simulink model "Control_simulation"  (R2016a)
settings: Solver=ode4  StartTime=0.0  StopTime=200  FixedStep=0.001  MaxStep=0.01  RelTol=1e-6
values from neighbouring files (symbols this model uses):
  float =     [waveglider.mat]
  floatABC =     [waveglider.mat]
  gliderABC =     [waveglider.mat]
undefined symbols (not defined in the file or in its folder): magnitude, RAO_Vel, sigbuilder_block
libraries: simulink_extras x8, simulink x5, marine_gnc x4, fuzblock x1, marine_hydro x1
(part 1 of 3)
settings Model: Creator=Administrator  LastModifiedBy=DELL

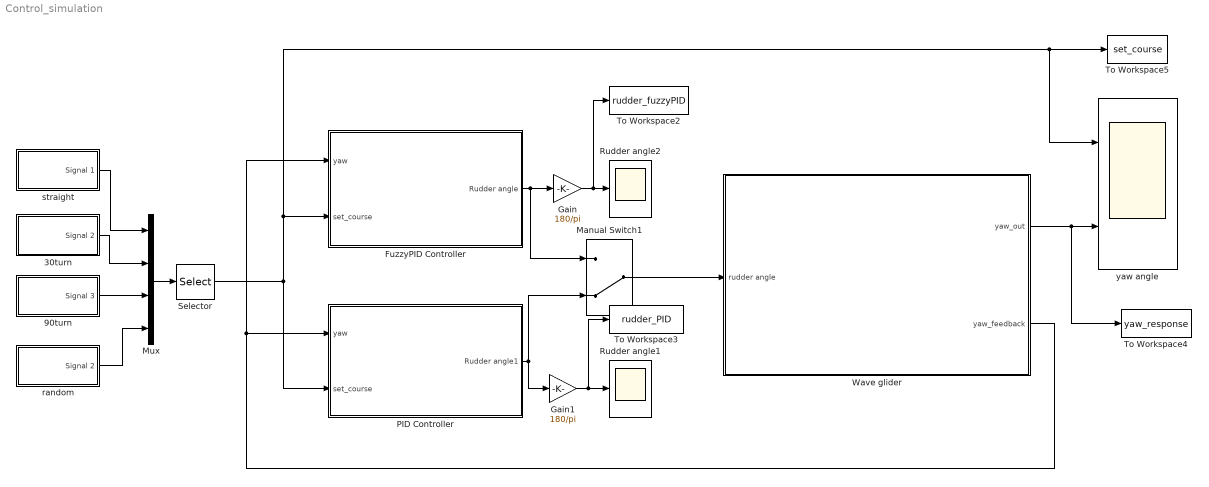
== system Control_simulation ==
  " yaw angle" : Scope  NumInputPorts=2
  30turn : Subsystem  Tag=STV Subsys  LoadFcn=sigbuilder_block('load');  StartFcn=sigbuilder_block('start');  StopFcn=sigbuilder_block('stop');  ClipboardFcn=sigbuilder_block('clipboard');  mask(Sigbuilder block){}
      mask help: Simulink:masks:SigbuilderBlock_MD
      mask init:
      | if ~strcmp(get_param(bdroot(gcbh),'SimulationStatus'),'stopped') tuvar = sigbuilder_block('maskInit'); end
      settings: CopyFcn=sigbuilder_block('copy');  DeleteFcn=sigbuilder_block('delete');  ModelCloseFcn=sigbuilder_block('modelClose');  PreSaveFcn=sigbuilder_block('preSave');  PauseFcn=sigbuilder_block('pause');  ContinueFcn=sigbuilder_block('continue');  NameChangeFcn=sigbuilder_block('namechange');  OpenFcn=sigbuilder_block('open',[6 105.75 1012.5 406.5 ]);  CloseFcn=sigbuilder_block('close');
      mask Display: plot(0, 0, 100, 100,[2, 2, 32, 32, 2], [68, 8, 8, 68, 68],[32, 2], [38, 38], [32, 19, 2],[53, 60, 44], [32, 17, 17, 2],[16, 16, 31, 31]);txt = getActiveGroup(gcbh);text(2, 100, txt,'verticalAlignment', 'top');
  90turn : Subsystem  Tag=STV Subsys  LoadFcn=sigbuilder_block('load');  StartFcn=sigbuilder_block('start');  StopFcn=sigbuilder_block('stop');  ClipboardFcn=sigbuilder_block('clipboard');  mask(Sigbuilder block){}
      mask help: Simulink:masks:SigbuilderBlock_MD
      mask init:
      | if ~strcmp(get_param(bdroot(gcbh),'SimulationStatus'),'stopped') tuvar = sigbuilder_block('maskInit'); end
      settings: CopyFcn=sigbuilder_block('copy');  DeleteFcn=sigbuilder_block('delete');  ModelCloseFcn=sigbuilder_block('modelClose');  PreSaveFcn=sigbuilder_block('preSave');  PauseFcn=sigbuilder_block('pause');  ContinueFcn=sigbuilder_block('continue');  NameChangeFcn=sigbuilder_block('namechange');  OpenFcn=sigbuilder_block('open',[6 16.5 1012.5 340.5 ]);  CloseFcn=sigbuilder_block('close');
      mask Display: plot(0, 0, 100, 100,[2, 2, 32, 32, 2], [68, 8, 8, 68, 68],[32, 2], [38, 38], [32, 19, 2],[53, 60, 44], [32, 17, 17, 2],[16, 16, 31, 31]);txt = getActiveGroup(gcbh);text(2, 100, txt,'verticalAlignment', 'top');
  FuzzyPID Controller : Subsystem
  Gain : Gain  Gain=180/pi
  Gain1 : Gain  Gain=180/pi
  Manual Switch1 : ManualSwitch  CurrentSetting=0
  Mux : Mux
  PID Controller : Subsystem
  Rudder angle1 : Scope
  Rudder angle2 : Scope
  Selector : Selector  InputPortWidth=4  IndexOptions=Index vector (dialog)  Indices=[4]  OutputSizes=1
  To Workspace2 : ToWorkspace  VariableName=rudder_fuzzyPID  SaveFormat=Timeseries  SampleTime=-1
  To Workspace3 : ToWorkspace  VariableName=rudder_PID  SaveFormat=Timeseries  SampleTime=-1
  To Workspace4 : ToWorkspace  VariableName=yaw_response  SaveFormat=Timeseries  SampleTime=-1
  To Workspace5 : ToWorkspace  VariableName=set_course  SaveFormat=Timeseries  SampleTime=-1
  Wave glider : Subsystem
  random : Subsystem  Tag=STV Subsys  LoadFcn=sigbuilder_block('load');  StartFcn=sigbuilder_block('start');  StopFcn=sigbuilder_block('stop');  ClipboardFcn=sigbuilder_block('clipboard');  mask(Sigbuilder block){}
      mask help: Simulink:masks:SigbuilderBlock_MD
      mask init:
      | if ~strcmp(get_param(bdroot(gcbh),'SimulationStatus'),'stopped') tuvar = sigbuilder_block('maskInit'); end
      settings: CopyFcn=sigbuilder_block('copy');  DeleteFcn=sigbuilder_block('delete');  ModelCloseFcn=sigbuilder_block('modelClose');  PreSaveFcn=sigbuilder_block('preSave');  PauseFcn=sigbuilder_block('pause');  ContinueFcn=sigbuilder_block('continue');  NameChangeFcn=sigbuilder_block('namechange');  OpenFcn=sigbuilder_block('open',[12 81 1006.5 339.75 ]);  CloseFcn=sigbuilder_block('close');
      mask Display: plot(0, 0, 100, 100,[2, 2, 32, 32, 2], [68, 8, 8, 68, 68],[32, 2], [38, 38], [32, 19, 2],[53, 60, 44], [32, 17, 17, 2],[16, 16, 31, 31]);txt = getActiveGroup(gcbh);text(2, 100, txt,'verticalAlignment', 'top');
  straight : Subsystem  Tag=STV Subsys  LoadFcn=sigbuilder_block('load');  StartFcn=sigbuilder_block('start');  StopFcn=sigbuilder_block('stop');  ClipboardFcn=sigbuilder_block('clipboard');  mask(Sigbuilder block){}
      mask help: Simulink:masks:SigbuilderBlock_MD
      mask init:
      | if ~strcmp(get_param(bdroot(gcbh),'SimulationStatus'),'stopped') tuvar = sigbuilder_block('maskInit'); end
      settings: CopyFcn=sigbuilder_block('copy');  DeleteFcn=sigbuilder_block('delete');  ModelCloseFcn=sigbuilder_block('modelClose');  PreSaveFcn=sigbuilder_block('preSave');  PauseFcn=sigbuilder_block('pause');  ContinueFcn=sigbuilder_block('continue');  NameChangeFcn=sigbuilder_block('namechange');  OpenFcn=sigbuilder_block('open',[106.5 139.5 1198.5 336.75 ]);  CloseFcn=sigbuilder_block('close');
      mask Display: plot(0, 0, 100, 100,[2, 2, 32, 32, 2], [68, 8, 8, 68, 68],[32, 2], [38, 38], [32, 19, 2],[53, 60, 44], [32, 17, 17, 2],[16, 16, 31, 31]);txt = getActiveGroup(gcbh);text(2, 100, txt,'verticalAlignment', 'top');
  wires:
  PID Controller/1(Rudder angle1) -> Gain1/1, Manual Switch1/2
  FuzzyPID Controller/1(Rudder angle) -> Manual Switch1/1, Gain/1
  Wave glider/1(yaw_out) -> To Workspace4/1, " yaw angle"/2
  Gain/1 -> To Workspace2/1, Rudder angle2/1
  Gain1/1 -> To Workspace3/1, Rudder angle1/1
  Mux/1 -> Selector/1
  Wave glider/2(yaw_feedback) -> FuzzyPID Controller/1(yaw), PID Controller/1(yaw)
  Selector/1 -> PID Controller/2(set_course), " yaw angle"/1, To Workspace5/1, FuzzyPID Controller/2(set_course)
  Manual Switch1/1 -> Wave glider/1(rudder angle)
  straight/1(Signal 1) -> Mux/1
  30turn/1(Signal 2) -> Mux/2
  90turn/1(Signal 3) -> Mux/3
  random/1(Signal 2) -> Mux/4

== system Control_simulation/30turn ==
  Demux : Demux  Tag=STV Demux  Outputs=1
  FromWs : FromWorkspace  Tag=STV FromWs  VariableName=tuvar  SampleTime=0
      SigBuilderData=|
      | common.afterFinalStr = 'Extrapolate'
      | common.sampleTime = 0
      | dataSet.timeRange = [0 500]
      | dataSet.name = 'Group 1'
      | sbobj.Groups.Name = 'Group 1'
      | sbobj.Groups.Signals.Name = 'Signal 2'
      | sbobj.Groups.Signals.XData = [0 50 50 100 100 150 150 200 200 250 250 300 300 350 350 400 400 450 450 500]
      | sbobj.Groups.Signals.YData = [0 0 30 30 -0.5 -0.5 30 30 0 0 30 30 0 0 30 30 0 0 30 30]
      | sbobj.Groups.TimeRange = [0 500]
  Signal 2 : Outport  Tag=STV Outport
  wires:
  FromWs/1 -> Demux/1
  Demux/1 -> Signal 2/1

== system Control_simulation/90turn ==
  Demux : Demux  Tag=STV Demux  Outputs=1
  FromWs : FromWorkspace  Tag=STV FromWs  VariableName=tuvar  SampleTime=0
      SigBuilderData=|
      | common.afterFinalStr = 'Extrapolate'
      | common.sampleTime = 0
      | dataSet.timeRange = [0 500]
      | dataSet.name = 'Group 1'
      | sbobj.Groups.Name = 'Group 1'
      | sbobj.Groups.Signals.Name = 'Signal 3'
      | sbobj.Groups.Signals.XData = [0 50 55 100 105 150 155 200 205 250 255 300 305 350.5 355 400 405 450 455 500]
      | sbobj.Groups.Signals.YData = [0 0 90 90 0 0 90 90 0 0 90 90 0 0 90 90 0 0 90 90]
      | sbobj.Groups.TimeRange = [0 500]
  Signal 3 : Outport  Tag=STV Outport
  wires:
  FromWs/1 -> Demux/1
  Demux/1 -> Signal 3/1

== system Control_simulation/FuzzyPID Controller ==
  yaw : Inport
  set_course : Inport  Port=2
  FuzzyPID Control : Subsystem
  Gain : Gain  Gain=pi/180
  Saturation : Saturate  UpperLimit=0.78  LowerLimit=-0.78
  Sum11 : Sum  Inputs=+-|  SaturateOnIntegerOverflow=on
  Rudder angle : Outport
  wires:
  FuzzyPID Control/1(Deta) -> Saturation/1
  Gain/1 -> Sum11/2
  set_course/1 -> Gain/1
  yaw/1 -> Sum11/1
  Sum11/1 -> FuzzyPID Control/1(e)
  Saturation/1 -> Rudder angle/1

== system Control_simulation/PID Controller ==
  yaw : Inport
  set_course : Inport  Port=2
  Gain : Gain  Gain=pi/180
  PID Controller : simulink/Continuous/PID Controller  Controller=PID  TimeDomain=Continuous-time  SampleTime=-1  IntegratorMethod=Forward Euler  FilterMethod=Forward Euler  Form=Parallel  UseFilter=on  ControllerParametersSource=internal  P=5.526  I=0.041  D=6.254  N=10  InitialConditionSource=internal  InitialConditionForIntegrator=0  InitialConditionForFilter=0  ExternalReset=none  LimitOutput=off  UpperSaturationLimit=inf  LowerSaturationLimit=-inf  LinearizeAsGain=on  AntiWindupMode=none  Kb=1  TrackingMode=off  Kt=1  PParamMin=[]  PParamMax=[]  IParamMin=[]  IParamMax=[]  DParamMin=[]  DParamMax=[]  NParamMin=[]  NParamMax=[]  KbParamMin=[]  KbParamMax=[]  KtParamMin=[]  KtParamMax=[]  POutMin=[]  POutMax=[]  IOutMin=[]  IOutMax=[]  DOutMin=[]  DOutMax=[]  NOutMin=[]  NOutMax=[]  KbOutMin=[]  KbOutMax=[]  KtOutMin=[]  KtOutMax=[]  IntegratorOutMin=[]  IntegratorOutMax=[]  FilterOutMin=[]  FilterOutMax=[]  SumOutMin=[]  SumOutMax=[]  SumI1OutMin=[]  SumI1OutMax=[]  SumI2OutMin=[]  SumI2OutMax=[]  SumI3OutMin=[]  SumI3OutMax=[]  SumDOutMin=[]  SumDOutMax=[]  SaturationOutMin=[]  SaturationOutMax=[]  IntegratorContinuousStateAttributes=''  IntegratorStateMustResolveToSignalObject=off  IntegratorRTWStateStorageClass=Auto  FilterContinuousStateAttributes=''  FilterStateMustResolveToSignalObject=off  FilterRTWStateStorageClass=Auto  DifferentiatorICPrevScaledInput=0  DifferentiatorOutMin=[]  DifferentiatorOutMax=[]
  Saturation : Saturate  UpperLimit=0.78  LowerLimit=-0.78
  Sum16 : Sum  Inputs=+-|  SaturateOnIntegerOverflow=on
  Rudder angle1 : Outport
  wires:
  yaw/1 -> Sum16/1
  set_course/1 -> Gain/1
  Sum16/1 -> PID Controller/1
  Gain/1 -> Sum16/2
  PID Controller/1 -> Saturation/1
  Saturation/1 -> Rudder angle1/1

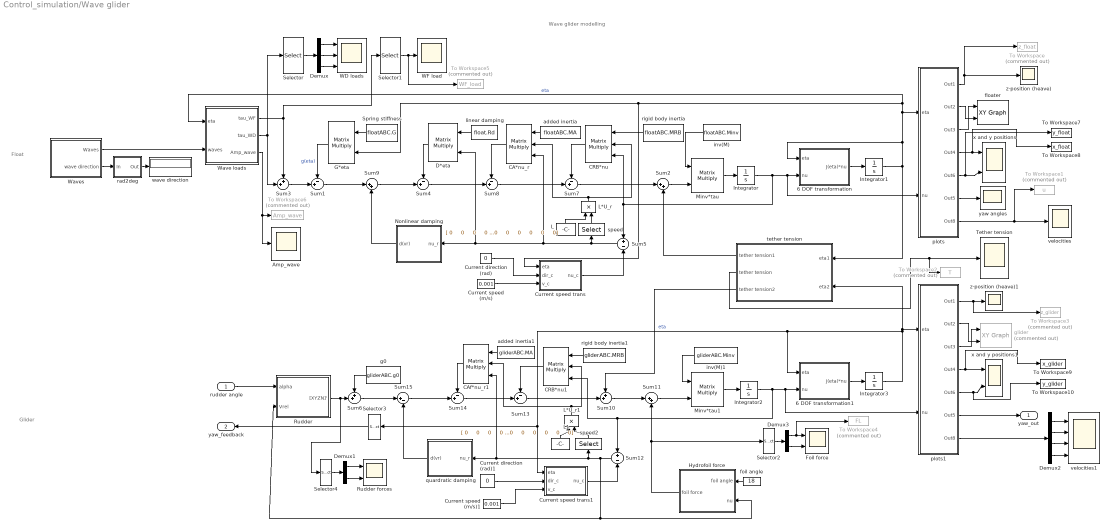
== system Control_simulation/Wave glider ==
  note: Float
  note: Wave glider modelling
  note: Glider
  rudder angle : Inport
  " yaw angles" : Scope
  6 DOF transformation : Subsystem  AncestorBlock=marine_gnc/Models/ Kinematics/6 DOF transformation
  6 DOF transformation1 : Subsystem  AncestorBlock=marine_gnc/Models/ Kinematics/6 DOF transformation
  Amp_wave : Scope
  CA*nu_r : Product  Inputs=3  Multiplication=Matrix(*)  RndMeth=Zero
  CAf*nu_r1 : Product  Inputs=3  Multiplication=Matrix(*)  RndMeth=Zero
  CRB*nu : Product  Inputs=3  Multiplication=Matrix(*)  RndMeth=Zero
  CRB*nu1 : Product  Inputs=3  Multiplication=Matrix(*)  RndMeth=Zero
  Current direction (rad) : Constant  Value=0
  Current direction (rad)1 : Constant  Value=0
  Current speed (m/s) : Constant  Value=0.001
  Current speed (m/s)1 : Constant  Value=0.001
  Current speed trans : Subsystem
  Current speed trans1 : Subsystem
  "D*eta " : Product  Multiplication=Matrix(*)  SaturateOnIntegerOverflow=on  OutDataTypeStr=Inherit: Same as first input
  Demux : Demux  Outputs=3
  Demux1 : Demux  Outputs=2
  Demux2 : Demux
  Demux3 : Demux  Outputs=2
  Foil force : Scope  NumInputPorts=2
  G*eta : Product  Multiplication=Matrix(*)  SaturateOnIntegerOverflow=on  OutDataTypeStr=Inherit: Same as first input
  Hydrofoil force : Subsystem
  Integrator : Integrator  InitialCondition=[0 0 0 0 0 0]
  Integrator1 : Integrator  InitialCondition=[0 0 0 0 0 0]
  Integrator2 : Integrator  InitialCondition=[0 0 0 0 0 0]
  Integrator3 : Integrator  InitialCondition=[0 0 6.2 0 0 0]
  L : Constant  Value=|
      | [ 0     0     0     0     0     0;   0     0     0     0     0     1;
      |      0     0     0     0    -1     0;	
      |      0     0     0     0     0     0	;
      |      0     0     0     0     0     0	
      | ;     0     0     0     0     0     0]
  L*U_r : Product  RndMeth=Zero
  L*U_r1 : Product  RndMeth=Zero
  L1 : Constant  Value=|
      | [ 0     0     0     0     0     0;   0     0     0     0     0     1;
      |      0     0     0     0    -1     0;	
      |      0     0     0     0     0     0	;
      |      0     0     0     0     0     0	
      | ;     0     0     0     0     0     0]
  Minv*tau : Product  Inputs=**  Multiplication=Matrix(*)  SaturateOnIntegerOverflow=on  OutDataTypeStr=Inherit: Same as first input
  Minv*tau1 : Product  Inputs=**  Multiplication=Matrix(*)  SaturateOnIntegerOverflow=on  OutDataTypeStr=Inherit: Same as first input
  Nonlinear damping : Subsystem
  Rudder : Subsystem  mask(Rudder Model){LCG=0.94, lamda=2, eks=7*pi/180, A=0.04, Cdc=0.8, CD0=0.008, rho=1025}
      mask prompts: LCG "LCG  [m]:"; A "Area (m^2):"; CD0 "CD0 (non-dim Drag @ zero angle of attack):"; rho "Water density  [Kg/m^3]:"
      mask help:
      | Model to generate forces and moments due to rudder action as a control surface.
      | Copyright (C) 2005 NTNU
      | Author: Tristan Perez
      mask Help:
      | This block gives the forces (N) and moments (Nm) in 4-DOF
      |  generated by the rudder.   The inputs of the block are the  effective  angle of attack  "alpha_eff"and  the average speed of the fluid over the rudder "V".
      | "LCG " is the longitudinal
      |  position of the centre of gravity
      | (distance from along the center line from the rudder stock to the CG.) "VCG" is the
      | vertical center of gravity (distance from the base line to GC.)
      | The lift generated is linear until  the stall angle is reached, where the lift saturates.
      | 
      | The units of the angles is in rad and the dCL/dalpha _e   shoudl have units of 1/rad.
  Rudder forces : Scope  NumInputPorts=2
  Selector : Selector  InputPortWidth=6  IndexOptions=Index vector (dialog)  Indices=[1 2 6]  OutputSizes=1
  Selector1 : Selector  InputPortWidth=6  IndexOptions=Index vector (dialog)  Indices=[3]  OutputSizes=1
  Selector2 : Selector  InputPortWidth=6  IndexOptions=Index vector (dialog)  Indices=[1 3]  OutputSizes=1
  Selector3 : Selector  InputPortWidth=6  IndexOptions=Index vector (dialog)  Indices=[6]  OutputSizes=1
  Selector4 : Selector  InputPortWidth=6  IndexOptions=Index vector (dialog)  Indices=[1 2]  OutputSizes=1
  Spring stiffness : Constant  Value=floatABC.G
  Sum{1,4,7..8,13..14} (6 alike) : Sum  Inputs=-+|  SaturateOnIntegerOverflow=on
  Sum10 : Sum  Inputs=++|  SaturateOnIntegerOverflow=on
  Sum11 : Sum  Inputs=|++  SaturateOnIntegerOverflow=on
  Sum12 : Sum  Inputs=+|-  SaturateOnIntegerOverflow=on
  Sum15 : Sum  Inputs=|+-  SaturateOnIntegerOverflow=on
  Sum2 : Sum  Inputs=|++  SaturateOnIntegerOverflow=on
  Sum3 : Sum  Inputs=++|  SaturateOnIntegerOverflow=on
  Sum5 : Sum  Inputs=+|-  SaturateOnIntegerOverflow=on
  Sum6 : Sum  Inputs=++|  SaturateOnIntegerOverflow=on
  Sum9 : Sum  Inputs=|++  SaturateOnIntegerOverflow=on
  Tether tension : Scope
  To Workspace : ToWorkspace  Commented=on  VariableName=z_float  SaveFormat=Timeseries  SampleTime=-1
  To Workspace1 : ToWorkspace  Commented=on  VariableName=u  SaveFormat=Timeseries  SampleTime=-1
  To Workspace10 : ToWorkspace  VariableName=y_glider  SaveFormat=Timeseries  SampleTime=-1
  To Workspace2 : ToWorkspace  Commented=on  VariableName=T  SaveFormat=Timeseries  SampleTime=-1
  To Workspace3 : ToWorkspace  Commented=on  VariableName=z_glider  SaveFormat=Timeseries  SampleTime=-1
  To Workspace4 : ToWorkspace  Commented=on  VariableName=FL  SaveFormat=Timeseries  SampleTime=-1
  To Workspace5 : ToWorkspace  Commented=on  VariableName=WF_load  SaveFormat=Timeseries  SampleTime=-1
  To Workspace6 : ToWorkspace  Commented=on  VariableName=Amp_wave  SaveFormat=Timeseries  SampleTime=-1
  To Workspace7 : ToWorkspace  VariableName=y_float  SaveFormat=Timeseries  SampleTime=-1
  To Workspace8 : ToWorkspace  VariableName=x_float  SaveFormat=Timeseries  SampleTime=-1
  To Workspace9 : ToWorkspace  VariableName=x_glider  SaveFormat=Timeseries  SampleTime=-1
  WD loads : Scope  NumInputPorts=3
  WF load : Scope
  Wave loads : Subsystem
  Waves : Subsystem  AncestorBlock=marine_gnc/Environment/Waves/Waves  mask(Waves){spectrum_type=Jonswap, disp_flag=on, plot_spectrum=off, plot_realization=off, hs=0.8, omega_peak=0.84, psi_mean=0, gamma=-1, spread=2, depth=inf, nfreq=20, ndir=1, energylim=0.005, freq_cutoff=3, dir_cutoff=0, rand_seed=0, rand_freq=on, rand_dir=on, Zeta_a=0, Omega=0, Phase=0, Wavenum=0, Psi=0}
      mask prompts: spectrum_type "Spectrum type"; disp_flag "Display initialization info in workspace window"; plot_spectrum "Plot spectrum"; plot_realization "Plot sea state realization (time-consuming)"; hs "Significant wave height Hs (m)"; omega_peak "Peak frequency omega_0 (rad/s)"; psi_mean "Mean wave direction (rad)"; gamma "Spectrum peakedness factor [1,7], 3.3 default, 0 for using DNV value"; spread "Wave spreading factor (1,2,3,4,5)"; depth "Average water depth (m), use inf for deep water"; nfreq "Number of frequencies in grid (recommended > 20)"; ndir "Number of directions in grid, 1 for long-crested waves"; energylim "Wave component energy limit [0 1] or number of waves (e.g. 50)"; freq_cutoff "Frequency cutoff factor [1.5, 5], default 3"; dir_cutoff "Direction cutoff [0, 3pi/8], default 0"; rand_seed "Random seed"; rand_freq "Random frequencies"; rand_dir "Random directions"; Zeta_a "Amplitude vector 'Zeta_a' (m)"; Omega "Frequency vector 'Omega' (rad/s)"; Phase "Phase vector 'Phase' (rad)"; Wavenum "Wavenumber vector 'Wavenum' (1/m)"; Psi "Direction vector 'Psi'  (rad)"
      mask help:
      | Calculate harmonic wave component parameters from a wave spectrum.
      | - Input one wave direction in the mask to get long-crested waves.
      | - Input zero peak frequency to get an expectation value from north sea statistical data.
      | - Input an integer > 1 for energylim to set the number of wave components fixed to nwaves = energylim.
      |
      | Copyright (C) 2004 NTNU
      | Author: Oyvind Notland Smogeli
      mask init:
      | if spectrum_type < 4
      | 	[Zeta_a, Omega, Phase, Wavenum, Psi] = Wave_init(spectrum_type, hs, omega_peak, psi_mean,...
      | 	gamma, spread, depth, nfreq, ndir, energylim, freq_cutoff, dir_cutoff, rand_freq, rand_dir,...
      | 	rand_seed, plot_spectrum, plot_realization, disp_flag);
      | end
      mask Help:
      | <font face="Arial">
      | <b>Project:</b> Marine Systems Simulator: MSS<br>
      | <br>
      | Define harmonic wave components describing the sea state by extracting
      | components from a given frequency and direction spectrum. The output from the
      | block is a bus containing the following wave parameter vectors:</font></p>
      | <p><font face="Arial"><b>Zeta_a</b>: Vector of harmonic wave amplitudes [m]<br>
      | <b>Omega: </b>Vector of harmonic wave frequencies [rad/s]<br>
      | <b>Phase: </b>Vector of harmonic wave phases (random) [rad]<br>
      | <b>Wavenum:</b> Vector of harmonic wave numbers [1/m]<br>
      | <b>Psi: </b>Vector of harmonic wave directions [rad]</font></p>
      | <p><font face="Arial">The time series of sea surface elevation Zeta(x,y,t) can
      | be obtained as</font></p>
      | <p><font face="Arial">Zeta(x,y,t) = Sum( Zeta_a(i)*cos(Omega(i)*t + Phase(i) - Wavenum(i)*(x*cos(Psi(i))
      | + y*sin(Psi(i)))) )</font></p>
      | <p><font face="Arial">where the sum is taken from i = 1 to i = n and n is the number of harmonic
      | wave components.</font></p>
      | <p>&nbsp;</p>
      | <p><font face="Arial">Input one wave direction to get long-crested waves.<br>
      | <br>
      | If the peak frequency is set to zero, then the peak frequency is obtained from
      | the sugnificant wave height usign a formula for the North Sea (Norsok):</font></p>
      | <p><font face="Arial">w0 = 2*pi/(4.883 + 2.68*Hs^0.54);</font></p>
      | 
      | <p>&nbsp;</p>
      | <p><font face="Arial">The energy limit (energylim) should be defined either as a positive factor
      | between 0 and 1, or as a positive integer. In the first case it will
      | discard all wave components with energy content less than this ratio of the
      | total energy content of the sea state. A recommended value is 0.005 or lower. In
      | the second case it will keep the nwaves = energylim most significant waves.</font></p>
      | <p>&nbsp;</p>
      | <p><font face="Arial">The wave elevation Zeta(x,y,t) at time t and at the coordinate (x,y) is found from the output vectors as:</font></p>
      | <p>&nbsp;</p>
      | <p><font face="Arial" color="#800000">References</font><ul>
      |   <li><font face="Arial">Sørensen, A.J. (2005) Lecture notes of TMR4240 &quot;Marine Cybernetics - Modelling and Control&quot;</font>
      |   <font face="Arial">Dept of Marine Technology NTNU.</font></li>
      |   <li><font face="Arial">Johannessen, K., T. S. Meling, S. Haver. Joint
      |   Distribution for Wind and<br>
      |   Waves in the Northern North Sea. IJOPE Vol. 12, No. 1, March 2002</font></li>
      |   <li>&nbsp;</li>
      |   </ul>
      | <p><font face="Arial">Johannessen, K., T. S. Meling, S. Haver. Joint
      | Distribution for Wind and<br>
      | Waves in the Northern North Sea. IJOPE Vol. 12, No. 1, March 2002</font><p>&nbsp;<p>
      |   <font face="Arial"><b>Author:</b> Øyvind Smogeli, September 2004 </font>
      | <p>&nbsp;</p>
      | <p>&nbsp;</p>
      mask TypeOptions spectrum_type: ITTC | Jonswap | Torsethaugen | Predefined waves
      mask Callback spectrum_type: Wave_callback;
  added inertia : Constant  Value=floatABC.MA
  added inertia1 : Constant  Value=gliderABC.MA
  floater : simulink/Sinks/XY Graph  xmin=-50  xmax=60  ymin=-50  ymax=60  st=-1
  foil angle : Constant  Value=18
  g0 : Constant  Value=gliderABC.g0
  glider : simulink/Sinks/XY Graph  Commented=on  xmin=0  xmax=30  ymin=0  ymax=30  st=-1
  inv(M) : Constant  Value=floatABC.Minv
  inv(M)1 : Constant  Value=gliderABC.Minv
  linear damping : Constant  Value=float.Rd
  plots : Subsystem
      mask Display: disp('time-series')
  plots1 : Subsystem
      mask Display: disp('time-series')
  quardratic damping : Subsystem
  rad2deg : Subsystem  AncestorBlock=marine_gnc/Utilities/Math Operations/Unit Conversion  mask(Unit Conversion){in=rad2deg}
      mask prompts: in "Convert"
      mask help:
      | Block to convert units. If the input in is a vector,
      | all the components are converted using the same conversion factor.
      |
      | Copyright (C) 2005 NTNU
      | Author:  Tristan Perez
      mask init:
      | if  in==1,
      | k=pi/180;
      | elseif  in==2,
      | k=180/pi;
      | elseif in==3,
      | k = .5145;
      | elseif in ==4,
      | k = 1/.5145;
      | 
      | end
      mask TypeOptions in: deg2rad | rad2deg | kt2m/sec | m/sec2 kt
  rigid body inertia : Constant  Value=floatABC.MRB
  rigid body inertia1 : Constant  Value=gliderABC.MRB
  speed : Selector  InputPortWidth=6  IndexOptions=Index vector (dialog)  Indices=[1]  OutputSizes=1
  speed2 : Selector  InputPortWidth=6  IndexOptions=Index vector (dialog)  Indices=[1]  OutputSizes=1
  tether tension : Subsystem
  velocities : Scope
  velocities1 : Scope  NumInputPorts=4
  wave direction : Display
  x and y positions : Scope  NumInputPorts=2
  x and y positions1 : Scope  NumInputPorts=2
  z-position (heave) : Scope
  z-position (heave)1 : Scope
  yaw_out : Outport
  yaw_feedback : Outport  Port=2
  wires:
  Demux2/1 -> velocities1/1
  plots1/1(Out1) -> To Workspace3/1, z-position (heave)1/1
  Demux/2 -> WD loads/2
  Waves/2(wave direction) -> rad2deg/1(In)
  Wave loads/3(Amp_wave) -> Amp_wave/1, To Workspace6/1
  plots/7(Out8) -> velocities/1, To Workspace1/1
  Sum3/1 -> Sum1/2
  tether tension/2(tether tension) -> To Workspace2/1, Tether tension/1
  rudder angle/1 -> Rudder/1("alpha ")
  tether tension/3(tether tension2) -> Sum10/1
  Demux3/2 -> Foil force/2
  plots1/5(Out6) -> To Workspace10/1, x and y positions1/2
  Sum10/1 -> Sum11/1
  Demux2/4 -> velocities1/4
  Demux/3 -> WD loads/3
  plots1/2(Out2) -> glider/2
  plots/5(Out6) -> To Workspace7/1, x and y positions/2
  Nonlinear damping/1(d(vr)) -> Sum9/2
  6 DOF transformation1/1(J(eta)*nu) -> Integrator3/1
  "D*eta "/1 -> Sum4/1
  Current direction (rad)1/1 -> Current speed trans1/2(dir_c)
  Selector2/1 -> Demux3/1
  L*U_r/1 -> CA*nu_r/2, CRB*nu/2
  rigid body inertia/1 -> CRB*nu/1
  CRB*nu1/1 -> Sum13/1
  Current speed (m/s)1/1 -> Current speed trans1/3(v_c)
  inv(M)/1 -> Minv*tau/1
  Minv*tau1/1 -> Integrator2/1
  Selector/1 -> Demux/1
  Sum15/1 -> Sum14/2
  Sum11/1 -> Minv*tau1/2
  Sum6/1 -> Sum15/1
  Sum9/1 -> Sum4/2
  CA*nu_r/1 -> Sum8/1
  CAf*nu_r1/1 -> Sum14/1
  added inertia1/1 -> CAf*nu_r1/1
  Sum12/1 -> quardratic damping/1(nu_r), CAf*nu_r1/3, speed2/1, Rudder/2(Vrel), Hydrofoil force/2(nu)
  Current speed trans/1(nu_c) -> Sum5/2
  Current speed (m/s)/1 -> Current speed trans/3(v_c)
  L*U_r1/1 -> CRB*nu1/2, CAf*nu_r1/2
  Sum7/1 -> Sum2/1
  speed/1 -> L*U_r/2
  Sum1/1 -> Sum9/1
  Rudder/1("[XYZN]'") -> Selector4/1, Sum6/2
  Current direction (rad)/1 -> Current speed trans/2(dir_c)
  L1/1 -> L*U_r1/1
  Minv*tau/1 -> Integrator/1
  rigid body inertia1/1 -> CRB*nu1/1
  plots/3(Out3) -> floater/1
  foil angle/1 -> Hydrofoil force/1(foil angle)
  plots/6(Out5) -> " yaw angles"/1
  Sum8/1 -> Sum7/2
  Sum2/1 -> Minv*tau/2
  Sum4/1 -> Sum8/2
  Current speed trans1/1(nu_c) -> Sum12/2
  linear damping/1 -> "D*eta "/1
  G*eta/1 -> Sum1/1  "g(eta)"
  rad2deg/1(Out) -> wave direction/1
  Hydrofoil force/1(foil force) -> Selector2/1, Sum11/2
  plots1/6(Out5) -> yaw_out/1
  Spring stiffness/1 -> G*eta/1
  Demux/1 -> WD loads/1
  Selector1/1 -> To Workspace5/1, WF load/1
  Integrator1/1 -> tether tension/1(eta1), plots/1(eta), Wave loads/1(eta), G*eta/2, Current speed trans/1(eta), 6 DOF transformation/1(eta)  "eta"
  6 DOF transformation/1(J(eta)*nu) -> Integrator1/1
  L/1 -> L*U_r/1
  Waves/1(Waves) -> Wave loads/2(waves)
  Sum13/1 -> Sum10/2
  speed2/1 -> L*U_r1/2
  Wave loads/2(tau_WD) -> Sum3/2, Selector/1
  Integrator3/1 -> tether tension/2(eta2), plots1/1(eta), Current speed trans1/1(eta), Selector3/1, 6 DOF transformation1/1(eta)  "eta"
  Demux2/3 -> velocities1/3
  plots1/4(Out4) -> x and y positions1/1, To Workspace9/1
  Demux3/1 -> To Workspace4/1, Foil force/1
  plots1/3(Out3) -> glider/1
  plots/1(Out1) -> To Workspace/1, z-position (heave)/1
  Demux2/2 -> velocities1/2
  tether tension/1(tether tension1) -> Sum2/2
  Sum5/1 -> Nonlinear damping/1(nu_r), "D*eta "/2, CA*nu_r/3, speed/1
  added inertia/1 -> CA*nu_r/1
  g0/1 -> Sum6/1
  Integrator/1 -> Sum5/1, CRB*nu/3, plots/2(nu), 6 DOF transformation/2(nu)
  Wave loads/1(tau_WF) -> Selector1/1, Sum3/1
  plots/2(Out2) -> floater/2
  inv(M)1/1 -> Minv*tau1/1
  Sum14/1 -> Sum13/2
  CRB*nu/1 -> Sum7/1
  plots1/7(Out8) -> Demux2/1
  quardratic damping/1(d(vr)) -> Sum15/2
  Integrator2/1 -> CRB*nu1/3, Sum12/1, plots1/2(nu), 6 DOF transformation1/2(nu)
  Selector3/1 -> yaw_feedback/1
  Demux1/2 -> Rudder forces/2
  Selector4/1 -> Demux1/1
  Demux1/1 -> Rudder forces/1
  plots/4(Out4) -> To Workspace8/1, x and y positions/1

== system Control_simulation/random ==
  Demux : Demux  Tag=STV Demux  Outputs=1
  FromWs : FromWorkspace  Tag=STV FromWs  VariableName=tuvar  SampleTime=0
      SigBuilderData=|
      | common.afterFinalStr = 'Extrapolate'
      | common.sampleTime = 0
      | dataSet.timeRange = [0 150]
      | dataSet.name = 'Group 1'
      | sbobj.Groups.Name = 'Group 1'
      | sbobj.Groups.Signals.Name = 'Signal 2'
      | sbobj.Groups.Signals.XData = [0 50 50 100 100 150]
      | sbobj.Groups.Signals.YData = [0 0 90 90 180 179.004016064]
      | sbobj.Groups.TimeRange = [0 150]
  Signal 2 : Outport  Tag=STV Outport
  wires:
  FromWs/1 -> Demux/1
  Demux/1 -> Signal 2/1

== system Control_simulation/straight ==
  Demux : Demux  Tag=STV Demux  Outputs=1
  FromWs : FromWorkspace  Tag=STV FromWs  VariableName=tuvar  SampleTime=0
      SigBuilderData=|
      | common.afterFinalStr = 'Extrapolate'
      | common.sampleTime = 0
      | dataSet.timeRange = [0 500]
      | dataSet.name = 'Group 1'
      | sbobj.Groups.Name = 'Group 1'
      | sbobj.Groups.Signals.Name = 'Signal 1'
      | sbobj.Groups.Signals.XData = [0 3.44827586207 6.89655172414 10.3448275862 13.7931034483 17.2413793103 20.6896551724 24.1379310345 27.5862068966 31.0344827586 34.4827586207 37.9310344828 41.3793103448 44.8275862069 48.275862069 51.724137931 55.1724137931 58.6206896552 62.0689655172 65.5172413793 68.9655172414 72.4137931034 75.8620689655 79.3103448276 82.7586206897 86.2068965517 89.6551724138 93.1034482759 96.5517241379 100 103.448275862 106.896551724 110.344827586 113.793103448 117.24137931 120.689655172 124.137931034 127.586206897 131.034482759 134.482758621 137.931034483 141.379310345 144.827586207 148.275862069 151.724137931 155.172413793 158.620689655 162.068965517 165.517241379 168.965517241 172.413793103 175.862068966 179.310344828 182.75862069 186.206896552 189.655172414 193.103448276 196.551724138 200 203.448275862 206.896551724 210.344827586 213.793103448 217.24137931 220.689655172 224.137931034 227.586206897 231.034482759 234.482758621 237.931034483 241.379310345 244.827586207 248.275862069 251.724137931 255.172413793 258.620689655 262.068965517 265.517241379 268.965517241 272.413793103 275.862068966 279.310344828 282.75862069 286.206896552 289.655172414 293.103448276 296.551724138 300 303.448275862 306.896551724 310.344827586 313.793103448 317.24137931 320.689655172 324.137931034 327.586206897 331.034482759 334.482758621 337.931034483 341.379310345 344.827586207 348.275862069 351.724137931 355.172413793 358.620689655 362.068965517 365.517241379 368.965517241 372.413793103 375.862068966 379.310344828 382.75862069 386.206896552 389.655172414 393.103448276 396.551724138 400 403.448275862 406.896551724 410.344827586 413.793103448 417.24137931 420.689655172 424.137931034 427.586206897 431.034482759 434.482758621 437.931034483 441.379310345 444.827586207 448.275862069 451.724137931 455.172413793 458.620689655 462.068965517 465.517241379 468.965517241 472.413793103 475.862068966 479.310344828 482.75862069 486.206896552 489.655172414 493.103448276 496.551724138 500]
      | sbobj.Groups.Signals.YData = [1 7.44911320633 13.5966730468 19.1552264558 23.8648616538 27.5053613334 29.9064997756 30.9560024155 30.6047956762 28.8693015945 25.8306699447 21.6309837656 ... (146 elements, 1x146)]
      | sbobj.Groups.TimeRange = [0 500]
  Signal 1 : Outport  Tag=STV Outport
  wires:
  FromWs/1 -> Demux/1
  Demux/1 -> Signal 1/1

== system Control_simulation/FuzzyPID Controller/FuzzyPID Control ==
  e : Inport
  D : Scope
  Demux : Demux  Outputs=2
  Derivative : Derivative
  Fuzzy Logic Controller : fuzblock/Fuzzy Logic  Controller  fis='FuzzyPID_revised.fis'
  Mux : Mux  Inputs=2
  P : Scope
  Subsystem : Subsystem
  Deta : Outport
  wires:
  Subsystem/1(Out1) -> Deta/1
  e/1 -> Mux/1, Subsystem/1(In1), Derivative/1
  Derivative/1 -> Mux/2
  Demux/1 -> P/1, Subsystem/2(In2)
  Demux/2 -> D/1, Subsystem/3(In4)
  Mux/1 -> Fuzzy Logic Controller/1
  Fuzzy Logic Controller/1 -> Demux/1

== system Control_simulation/Wave glider/6 DOF transformation ==
  note: omega
  note: v
  note: Theta
  eta : Inport
  nu : Inport  Port=2
  Euler angles to rotation matrix1 : Subsystem  AncestorBlock=marine_gnc/Models/ Kinematics/Euler angles to rotation matrix  mask(Euler2R){}
      mask help: Determine the 3-by-3 rotation matrix from the Euler angles (roll, pitch, yaw) using the zyx convention.
      mask Display:
      | port_label('input',1,'theta')
      | port_label('output',1,'R')
  Euler angles to attitude transformation matrix : marine_gnc/Models/ Kinematics/Euler angles to attitude transformation matrix
  Mux : Mux  Inputs=2
  Product : Product  Inputs=**  Multiplication=Matrix(*)  SaturateOnIntegerOverflow=on  OutDataTypeStr=Inherit: Same as first input
  Product1 : Product  Inputs=**  Multiplication=Matrix(*)  SaturateOnIntegerOverflow=on  OutDataTypeStr=Inherit: Same as first input
  Selector : Selector  InputPortWidth=6  IndexOptions=Index vector (dialog)  Indices=[4 5 6]  OutputSizes=1
  Selector1 : Selector  InputPortWidth=6  IndexOptions=Index vector (dialog)  Indices=[1 2 3]  OutputSizes=1
  Selector2 : Selector  InputPortWidth=6  IndexOptions=Index vector (dialog)  Indices=[4 5 6]  OutputSizes=1
  J(eta)*nu : Outport
  wires:
  Product1/1 -> Mux/2
  Mux/1 -> J(eta)*nu/1
  Product/1 -> Mux/1
  Euler angles to attitude transformation matrix/1 -> Product1/1
  Selector2/1 -> Product1/2
  Selector1/1 -> Product/2
  nu/1 -> Selector2/1, Selector1/1
  Euler angles to rotation matrix1/1(Rzyx) -> Product/1
  eta/1 -> Selector/1
  Selector/1 -> Euler angles to attitude transformation matrix/1, Euler angles to rotation matrix1/1(theta)

== system Control_simulation/Wave glider/6 DOF transformation1 ==
  note: omega
  note: v
  note: Theta
  eta : Inport
  nu : Inport  Port=2
  Euler angles to rotation matrix1 : Subsystem  AncestorBlock=marine_gnc/Models/ Kinematics/Euler angles to rotation matrix  mask(Euler2R){}
      mask help: Determine the 3-by-3 rotation matrix from the Euler angles (roll, pitch, yaw) using the zyx convention.
      mask Display:
      | port_label('input',1,'theta')
      | port_label('output',1,'R')
  Euler angles to attitude transformation matrix : marine_gnc/Models/ Kinematics/Euler angles to attitude transformation matrix
  Mux : Mux  Inputs=2
  Product : Product  Inputs=**  Multiplication=Matrix(*)  SaturateOnIntegerOverflow=on  OutDataTypeStr=Inherit: Same as first input
  Product1 : Product  Inputs=**  Multiplication=Matrix(*)  SaturateOnIntegerOverflow=on  OutDataTypeStr=Inherit: Same as first input
  Selector : Selector  InputPortWidth=6  IndexOptions=Index vector (dialog)  Indices=[4 5 6]  OutputSizes=1
  Selector1 : Selector  InputPortWidth=6  IndexOptions=Index vector (dialog)  Indices=[1 2 3]  OutputSizes=1
  Selector2 : Selector  InputPortWidth=6  IndexOptions=Index vector (dialog)  Indices=[4 5 6]  OutputSizes=1
  J(eta)*nu : Outport
  wires:
  Product1/1 -> Mux/2
  Mux/1 -> J(eta)*nu/1
  Product/1 -> Mux/1
  Euler angles to attitude transformation matrix/1 -> Product1/1
  Selector2/1 -> Product1/2
  Selector1/1 -> Product/2
  nu/1 -> Selector2/1, Selector1/1
  Euler angles to rotation matrix1/1(Rzyx) -> Product/1
  eta/1 -> Selector/1
  Selector/1 -> Euler angles to attitude transformation matrix/1, Euler angles to rotation matrix1/1(theta)

== system Control_simulation/Wave glider/Current speed trans ==
  eta : Inport
  dir_c : Inport  Port=2
  v_c : Inport  Port=3
  Sum : Sum  Inputs=|+-
  current1 : Subsystem
  yaw : Selector  InputPortWidth=6  IndexOptions=Index vector (dialog)  Indices=[6]  OutputSizes=1
  nu_c : Outport
  wires:
  dir_c/1 -> Sum/1
  v_c/1 -> current1/2(V_c(m/s))
  yaw/1 -> Sum/2
  current1/1(nu_c) -> nu_c/1
  Sum/1 -> current1/1(beta_c(rad))
  eta/1 -> yaw/1

== system Control_simulation/Wave glider/Current speed trans1 ==
  eta : Inport
  dir_c : Inport  Port=2
  v_c : Inport  Port=3
  Sum : Sum  Inputs=|+-
  current1 : Subsystem
  yaw : Selector  InputPortWidth=6  IndexOptions=Index vector (dialog)  Indices=[6]  OutputSizes=1
  nu_c : Outport
  wires:
  dir_c/1 -> Sum/1
  v_c/1 -> current1/2(V_c(m/s))
  yaw/1 -> Sum/2
  current1/1(nu_c) -> nu_c/1
  Sum/1 -> current1/1(beta_c(rad))
  eta/1 -> yaw/1

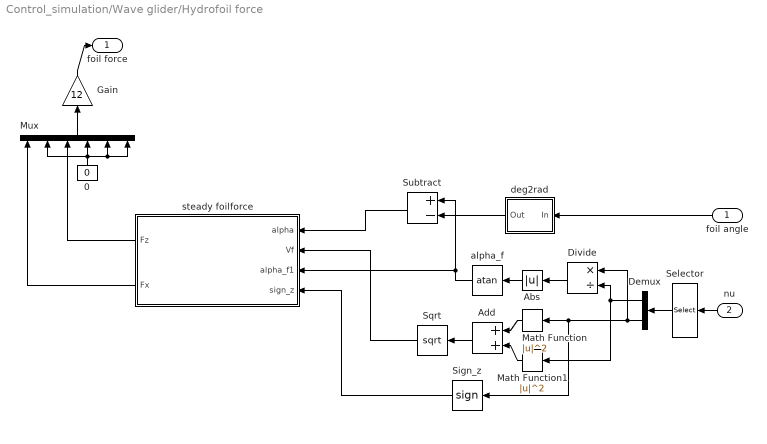
== system Control_simulation/Wave glider/Hydrofoil force ==
  foil angle : Inport
  nu : Inport  Port=2
  0 : Constant  Value=0
  Abs : Abs
  Add : Sum
  Demux : Demux  Outputs=2
  Divide : Product  Inputs=*/
  Gain : Gain  Gain=12
  Math Function : Math  Operator=magnitude^2  SaturateOnIntegerOverflow=on
  Math Function1 : Math  Operator=magnitude^2  SaturateOnIntegerOverflow=on
  Mux : Mux  Inputs=6
  Selector : Selector  InputPortWidth=6  IndexOptions=Index vector (dialog)  Indices=[1 3]  OutputSizes=1
  Sign_z : Signum
  Sqrt : Sqrt  SaturateOnIntegerOverflow=on
  Subtract : Sum  Inputs=+-
  alpha_f : Trigonometry  Operator=atan
  deg2rad : Subsystem  AncestorBlock=marine_gnc/Utilities/Math Operations/Unit Conversion  mask(Unit Conversion){in=deg2rad}
      mask prompts: in "Convert"
      mask help:
      | Block to convert units. If the input in is a vector,
      | all the components are converted using the same conversion factor.
      |
      | Copyright (C) 2005 NTNU
      | Author:  Tristan Perez
      mask init:
      | if  in==1,
      | k=pi/180;
      | elseif  in==2,
      | k=180/pi;
      | elseif in==3,
      | k = .5145;
      | elseif in ==4,
      | k = 1/.5145;
      | 
      | end
      mask TypeOptions in: deg2rad | rad2deg | kt2m/sec | m/sec2 kt
  steady foilforce : Subsystem  mask{Cdc=0.6, lamda=2, CD0=0.008, eks=7*pi/180, rho=1025, A=0.113}
  foil force : Outport
  wires:
  steady foilforce/1(Fz) -> Mux/3
  Mux/1 -> Gain/1
  0/1 -> Mux/6, Mux/5, Mux/2, Mux/4
  steady foilforce/2(Fx) -> Mux/1
  foil angle/1 -> deg2rad/1(In)
  nu/1 -> Selector/1
  Gain/1 -> foil force/1
  Selector/1 -> Demux/1
  Demux/1 -> Divide/2, Math Function1/1
  Demux/2 -> Sign_z/1, Math Function/1, Divide/1
  Divide/1 -> Abs/1
  Subtract/1 -> steady foilforce/1(alpha)
  alpha_f/1 -> steady foilforce/3(alpha_f1), Subtract/1
  deg2rad/1(Out) -> Subtract/2
  Math Function/1 -> Add/1
  Math Function1/1 -> Add/2
  Add/1 -> Sqrt/1
  Sqrt/1 -> steady foilforce/2("Vf ")
  Sign_z/1 -> steady foilforce/4(sign_z)
  Abs/1 -> alpha_f/1

== system Control_simulation/Wave glider/Nonlinear damping ==
  nu_r : Inport
  Cross-flow drag and surge resistance : marine_hydro/Hydro Library/Cross-flow drag and surge resistance  N=20  Lpp=2.1  CD=0.7  Cx=0.6  Ax=0.09  Ay=0.3  rho_w=1025
  Mux : Mux  Inputs=6
  zero : Constant  Value=0
  d(vr) : Outport
  wires:
  zero/1 -> Mux/5, Mux/3, Mux/4
  Cross-flow drag and surge resistance/3 -> Mux/6
  Cross-flow drag and surge resistance/2 -> Mux/2
  Cross-flow drag and surge resistance/1 -> Mux/1
  nu_r/1 -> Cross-flow drag and surge resistance/1
  Mux/1 -> d(vr)/1

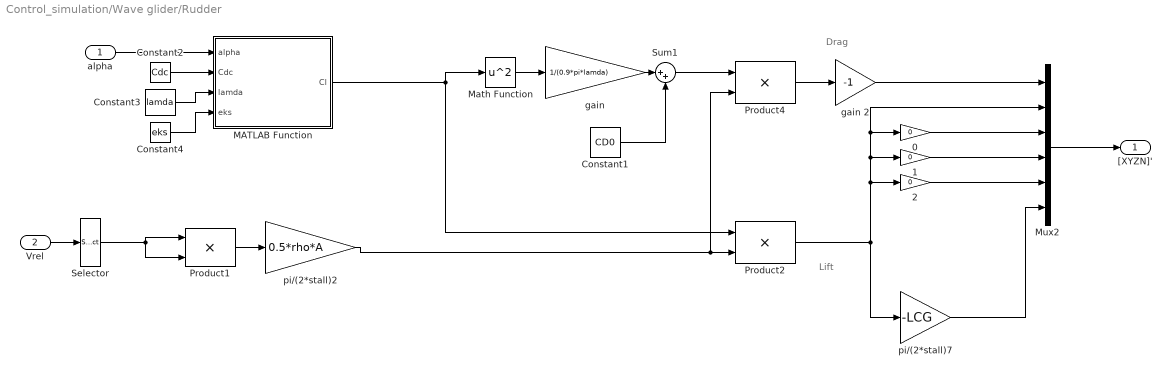
== system Control_simulation/Wave glider/Rudder ==
  note: Lift
  note: Drag
  "alpha " : Inport
  Vrel : Inport  Port=2
  0 : Gain  Gain=0  SaturateOnIntegerOverflow=on  OutDataTypeStr=Inherit: Same as input  ParamDataTypeStr=Inherit: Same as input
  1 : Gain  Gain=0  SaturateOnIntegerOverflow=on  OutDataTypeStr=Inherit: Same as input  ParamDataTypeStr=Inherit: Same as input
  2 : Gain  Gain=0  SaturateOnIntegerOverflow=on  OutDataTypeStr=Inherit: Same as input  ParamDataTypeStr=Inherit: Same as input
  Constant1 : Constant  Value=CD0
  Constant2 : Constant  Value=Cdc
  Constant3 : Constant  Value=lamda
  Constant4 : Constant  Value=eks
  MATLAB Function : MATLAB Function  TreatAsAtomicUnit=on
  Math Function : Math  Operator=square  SaturateOnIntegerOverflow=on
  Mux2 : Mux  Inputs=6
  Product1 : Product  Inputs=**  SaturateOnIntegerOverflow=on  InputSameDT=on  OutDataTypeStr=Inherit: Same as first input
  Product2 : Product  SaturateOnIntegerOverflow=on  InputSameDT=on  OutDataTypeStr=Inherit: Same as first input
  Product4 : Product  SaturateOnIntegerOverflow=on  InputSameDT=on  OutDataTypeStr=Inherit: Same as first input
  Selector : Selector  InputPortWidth=6  IndexOptions=Index vector (dialog)  Indices=[1]  OutputSizes=1
  Sum1 : Sum  Inputs=|++  SaturateOnIntegerOverflow=on  InputSameDT=on  OutDataTypeStr=Inherit: Same as first input
  "gain " : Gain  Gain=1/(0.9*pi*lamda)  SaturateOnIntegerOverflow=on  OutDataTypeStr=Inherit: Same as input  ParamDataTypeStr=Inherit: Same as input
  gain 2 : Gain  Gain=-1  SaturateOnIntegerOverflow=on  OutDataTypeStr=Inherit: Same as input  ParamDataTypeStr=Inherit: Same as input
  pi/(2*stall)2 : Gain  Gain=0.5*rho*A  SaturateOnIntegerOverflow=on  OutDataTypeStr=Inherit: Same as input  ParamDataTypeStr=Inherit: Same as input
  pi/(2*stall)7 : Gain  Gain=-LCG  SaturateOnIntegerOverflow=on  OutDataTypeStr=Inherit: Same as input  ParamDataTypeStr=Inherit: Same as input
  "[XYZN]'" : Outport
  wires:
  Product1/1 -> pi/(2*stall)2/1
  Vrel/1 -> Selector/1
  Constant1/1 -> Sum1/2
  "gain "/1 -> Sum1/1
  Math Function/1 -> "gain "/1
  Sum1/1 -> Product4/1
  pi/(2*stall)2/1 -> Product2/2, Product4/2
  Product4/1 -> gain 2/1
  gain 2/1 -> Mux2/1
  Mux2/1 -> "[XYZN]'"/1
  0/1 -> Mux2/3
  Product2/1 -> 2/1, 1/1, Mux2/2, 0/1, pi/(2*stall)7/1
  pi/(2*stall)7/1 -> Mux2/6
  MATLAB Function/1(Cl) -> Product2/1, Math Function/1
  "alpha "/1 -> MATLAB Function/1(alpha)
  1/1 -> Mux2/4
  2/1 -> Mux2/5
  Constant2/1 -> MATLAB Function/2(Cdc)
  Constant3/1 -> MATLAB Function/3(lamda)
  Constant4/1 -> MATLAB Function/4(eks)
  Selector/1 -> Product1/2, Product1/1
